simulink subsystem "tireTemp"  (R2022b)
settings: Solver=VariableStepAuto  StartTime=0.0  StopTime=10.0  RelTol=1e-3
libraries: tires x12
settings Model: Creator=serga  LastModifiedBy=serga

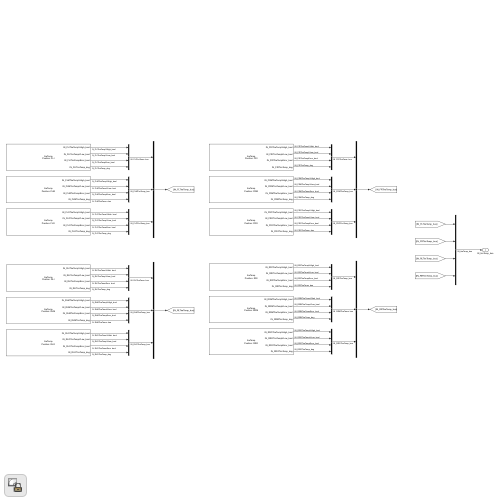
[thumbnail: Simulink's stored preview of the top-level diagram]
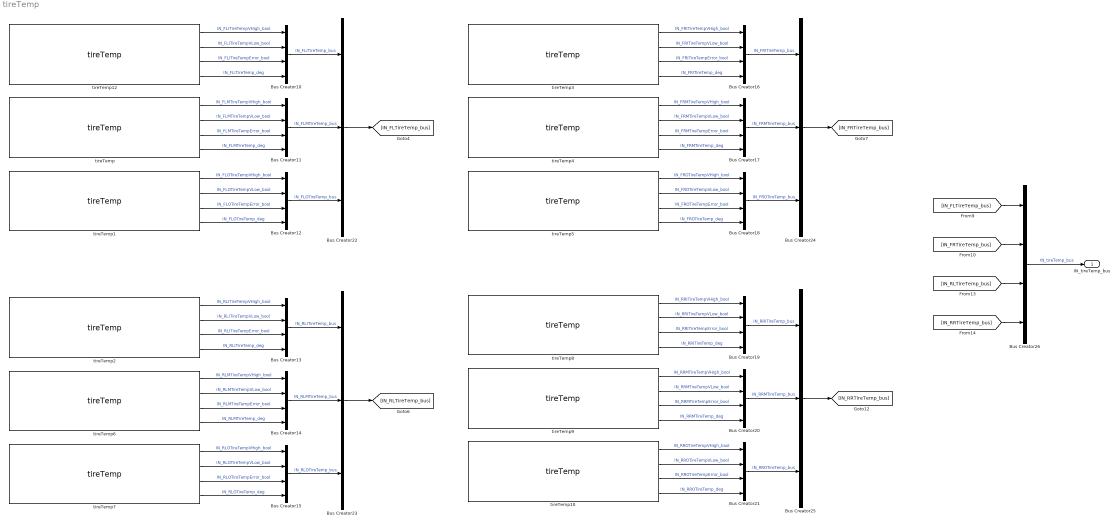
== system tireTemp ==
  Bus Creator{10..21,26} (13 alike) : BusCreator  Inputs=4
  Bus Creator{22..25} (4 alike) : BusCreator  Inputs=3
  tireTemp : tires/tireTemp  pos='FLM'
  tireTemp1 : tires/tireTemp  pos='FLO'
  tireTemp10 : tires/tireTemp  pos='RRO'
  tireTemp12 : tires/tireTemp  pos='FLI'
  tireTemp2 : tires/tireTemp  pos='RLI'
  tireTemp3 : tires/tireTemp  pos='FRI'
  tireTemp4 : tires/tireTemp  pos='FRM'
  tireTemp5 : tires/tireTemp  pos='FRO'
  tireTemp6 : tires/tireTemp  pos='RLM'
  tireTemp7 : tires/tireTemp  pos='RLO'
  tireTemp8 : tires/tireTemp  pos='RRI'
  tireTemp9 : tires/tireTemp  pos='RRM'
  IN_tireTemp_bus : Outport
  wires:
  tireTemp6/3 -> Bus Creator14/3  "IN_RLMTireTempError_bool"
  tireTemp/4 -> Bus Creator11/4  "IN_FLMTireTemp_deg"
  Bus Creator13/1 -> Bus Creator23/1  "IN_RLITireTemp_bus"
  Bus Creator12/1 -> Bus Creator22/3  "IN_FLOTireTemp_bus"
  Bus Creator25/1 -> [IN_RRTireTemp_bus]
  tireTemp8/1 -> Bus Creator19/1  "IN_RRITireTempVHigh_bool"
  tireTemp8/4 -> Bus Creator19/4  "IN_RRITireTemp_deg"
  tireTemp4/3 -> Bus Creator17/3  "IN_FRMTireTempError_bool"
  tireTemp7/1 -> Bus Creator15/1  "IN_RLOTireTempVHigh_bool"
  tireTemp10/1 -> Bus Creator21/1  "IN_RROTireTempVHigh_bool"
  tireTemp8/3 -> Bus Creator19/3  "IN_RRITireTempError_bool"
  Bus Creator20/1 -> Bus Creator25/2  "IN_RRMTireTemp_bus"
  Bus Creator14/1 -> Bus Creator23/2  "IN_RLMTireTemp_bus"
  tireTemp5/3 -> Bus Creator18/3  "IN_FROTireTempError_bool"
  [IN_RRTireTemp_bus] -> Bus Creator26/4
  [IN_RLTireTemp_bus] -> Bus Creator26/3
  Bus Creator19/1 -> Bus Creator25/1  "IN_RRITireTemp_bus"
  tireTemp5/4 -> Bus Creator18/4  "IN_FROTireTemp_deg"
  Bus Creator23/1 -> [IN_RLTireTemp_bus]
  tireTemp9/1 -> Bus Creator20/1  "IN_RRMTireTempVHigh_bool"
  [IN_FRTireTemp_bus] -> Bus Creator26/2
  Bus Creator17/1 -> Bus Creator24/2  "IN_FRMTireTemp_bus"
  Bus Creator15/1 -> Bus Creator23/3  "IN_RLOTireTemp_bus"
  Bus Creator22/1 -> [IN_FLTireTemp_bus]
  tireTemp12/3 -> Bus Creator10/3  "IN_FLITireTempError_bool"
  Bus Creator18/1 -> Bus Creator24/3  "IN_FROTireTemp_bus"
  tireTemp/3 -> Bus Creator11/3  "IN_FLMTireTempError_bool"
  Bus Creator16/1 -> Bus Creator24/1  "IN_FRITireTemp_bus"
  Bus Creator24/1 -> [IN_FRTireTemp_bus]
  tireTemp9/4 -> Bus Creator20/4  "IN_RRMTireTemp_deg"
  tireTemp9/2 -> Bus Creator20/2  "IN_RRMTireTempVLow_bool"
  tireTemp2/4 -> Bus Creator13/4  "IN_RLITireTemp_deg"
  Bus Creator21/1 -> Bus Creator25/3  "IN_RROTireTemp_bus"
  Bus Creator10/1 -> Bus Creator22/1  "IN_FLITireTemp_bus"
  tireTemp10/4 -> Bus Creator21/4  "IN_RROTireTemp_deg"
  tireTemp3/3 -> Bus Creator16/3  "IN_FRITireTempError_bool"
  tireTemp5/1 -> Bus Creator18/1  "IN_FROTireTempVHigh_bool"
  tireTemp2/2 -> Bus Creator13/2  "IN_RLITireTempVLow_bool"
  tireTemp8/2 -> Bus Creator19/2  "IN_RRITireTempVLow_bool"
  tireTemp1/4 -> Bus Creator12/4  "IN_FLOTireTemp_deg"
  tireTemp1/3 -> Bus Creator12/3  "IN_FLOTireTempError_bool"
  tireTemp4/2 -> Bus Creator17/2  "IN_FRMTireTempVLow_bool"
  tireTemp1/2 -> Bus Creator12/2  "IN_FLOTireTempVLow_bool"
  tireTemp12/4 -> Bus Creator10/4  "IN_FLITireTemp_deg"
  tireTemp/2 -> Bus Creator11/2  "IN_FLMTireTempVLow_bool"
  tireTemp/1 -> Bus Creator11/1  "IN_FLMTireTempVHigh_bool"
  tireTemp6/1 -> Bus Creator14/1  "IN_RLMTireTempVHigh_bool"
  tireTemp12/1 -> Bus Creator10/1  "IN_FLITireTempVHigh_bool"
  tireTemp3/4 -> Bus Creator16/4  "IN_FRITireTemp_deg"
  tireTemp3/2 -> Bus Creator16/2  "IN_FRITireTempVLow_bool"
  tireTemp10/2 -> Bus Creator21/2  "IN_RROTireTempVLow_bool"
  tireTemp1/1 -> Bus Creator12/1  "IN_FLOTireTempVHigh_bool"
  tireTemp9/3 -> Bus Creator20/3  "IN_RRMTireTempError_bool"
  tireTemp6/4 -> Bus Creator14/4  "IN_RLMTireTemp_deg"
  tireTemp5/2 -> Bus Creator18/2  "IN_FROTireTempVLow_bool"
  tireTemp4/1 -> Bus Creator17/1  "IN_FRMTireTempVHigh_bool"
  [IN_FLTireTemp_bus] -> Bus Creator26/1
  tireTemp4/4 -> Bus Creator17/4  "IN_FRMTireTemp_deg"
  Bus Creator11/1 -> Bus Creator22/2  "IN_FLMTireTemp_bus"
  tireTemp12/2 -> Bus Creator10/2  "IN_FLITireTempVLow_bool"
  tireTemp7/3 -> Bus Creator15/3  "IN_RLOTireTempError_bool"
  tireTemp7/2 -> Bus Creator15/2  "IN_RLOTireTempVLow_bool"
  tireTemp2/1 -> Bus Creator13/1  "IN_RLITireTempVHigh_bool"
  tireTemp10/3 -> Bus Creator21/3  "IN_RROTireTempError_bool"
  tireTemp3/1 -> Bus Creator16/1  "IN_FRITireTempVHigh_bool"
  tireTemp7/4 -> Bus Creator15/4  "IN_RLOTireTemp_deg"
  tireTemp6/2 -> Bus Creator14/2  "IN_RLMTireTempVLow_bool"
  tireTemp2/3 -> Bus Creator13/3  "IN_RLITireTempError_bool"
  Bus Creator26/1 -> IN_tireTemp_bus/1  "IN_tireTemp_bus"
